simulink model "Low_Pass_Filter"  (R2022b)
settings: Solver=VariableStepAuto  StartTime=0.0  StopTime=0.5  MaxStep=0.00001  RelTol=1e-3
settings Model: Creator=Administrator  LastModifiedBy=Administrator

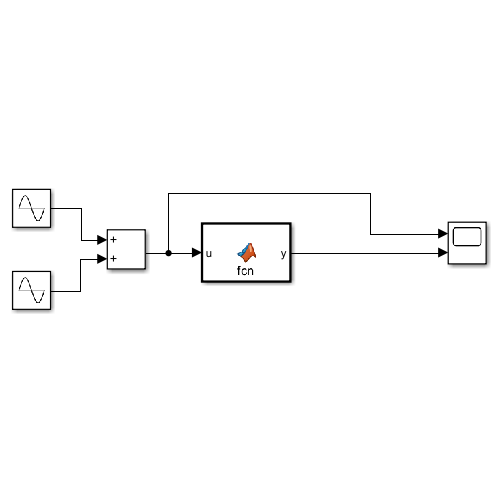
[thumbnail: Simulink's stored preview of the top-level diagram]
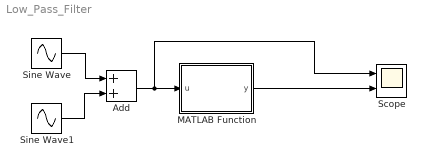
== system Low_Pass_Filter ==
  Add : Sum
  MATLAB Function : MATLAB Function  TreatAsAtomicUnit=on
  Scope : Scope  NumInputPorts=2
  Sine Wave : Sin  Amplitude=2  Frequency=100*2*pi  SampleTime=0
  Sine Wave1 : Sin  Amplitude=0.3  Frequency=10000*2*pi  SampleTime=0
  wires:
  Sine Wave/1 -> Add/1
  Sine Wave1/1 -> Add/2
  MATLAB Function/1(y) -> Scope/2
  Add/1 -> Scope/1, MATLAB Function/1(u)

== matlab function Low_Pass_Filter/MATLAB Function ==
  data: u input; y output
function y = fcn(u)
%#codegen
persistent yk yk_1 Tsc wc
if isempty(yk)
    yk = 0;
    yk_1 = 0;
    Tsc =0.0001;
    wc =100;
end
 sum = (1+wc*Tsc);
    alpha = 1 / sum;
    beta = wc*Tsc / sum;
    yk = alpha*yk_1 + beta*u;
    yk_1 = yk;
y = yk;
